simulink library "Junction_Lib"  (R2019a)
settings: Solver=VariableStepAuto  StartTime=0.0  StopTime=10.0  RelTol=1e-3
settings Model: Creator=martin  LastModifiedBy=martin

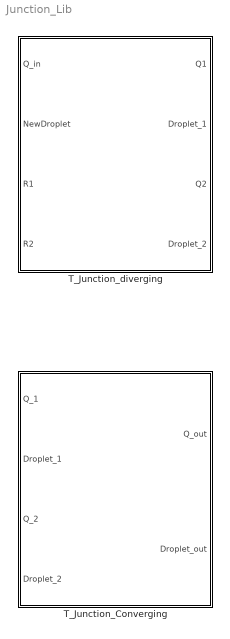
== system Junction_Lib ==
  T_Junction_Converging : Subsystem
  T_Junction_diverging : Subsystem

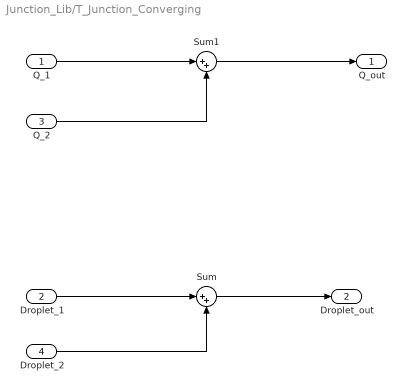
== system Junction_Lib/T_Junction_Converging ==
  Q_1 : Inport
  Droplet_1 : Inport  Port=2
  Q_2 : Inport  Port=3
  Droplet_2 : Inport  Port=4
  Sum : Sum  Inputs=|++
  Sum1 : Sum  Inputs=|++
  Q_out : Outport
  Droplet_out : Outport  Port=2
  wires:
  Droplet_1/1 -> Sum/1
  Sum/1 -> Droplet_out/1
  Droplet_2/1 -> Sum/2
  Q_1/1 -> Sum1/1
  Sum1/1 -> Q_out/1
  Q_2/1 -> Sum1/2

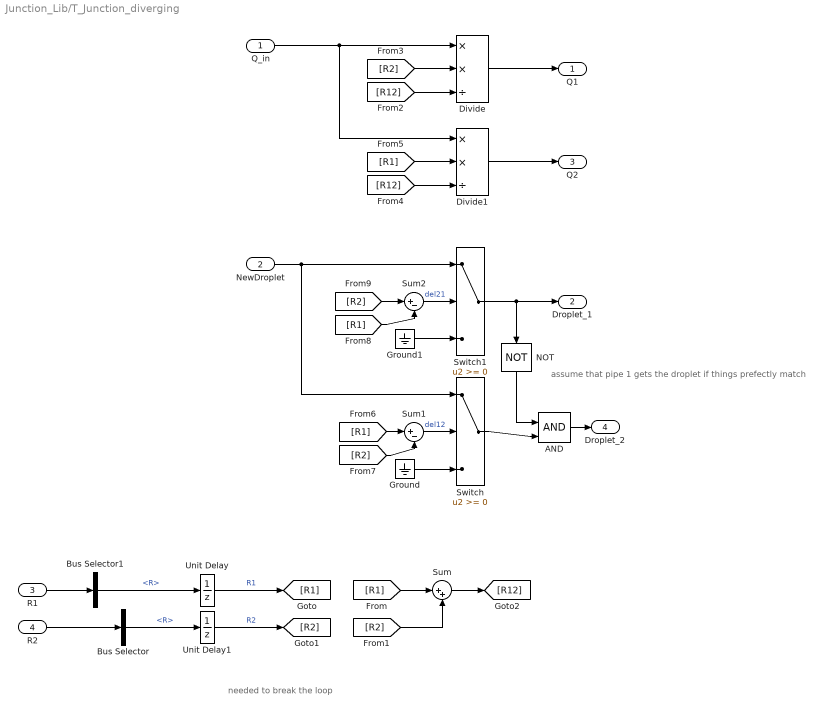
== system Junction_Lib/T_Junction_diverging ==
  note: assume that pipe 1 gets the droplet if things prefectly match
  note: needed to break the loop
  Q_in : Inport
  NewDroplet : Inport  Port=2
  R1 : Inport  Port=3
  R2 : Inport  Port=4
  AND : Logic  IconShape=distinctive  AllPortsSameDT=off  OutDataTypeStr=boolean
  Bus Selector : BusSelector  OutputSignals=R
  Bus Selector1 : BusSelector  OutputSignals=R
  Divide : Product  Inputs=**/
  Divide1 : Product  Inputs=**/
  Ground : Ground
  Ground1 : Ground
  NOT : Logic  Operator=NOT  IconShape=distinctive  AllPortsSameDT=off  OutDataTypeStr=boolean
  Sum : Sum  Inputs=|++
  Sum1 : Sum  Inputs=|+-
  Sum2 : Sum  Inputs=|+-
  Switch : Switch
  Switch1 : Switch
  Unit Delay : UnitDelay  SampleTime=-1  HasFrameUpgradeWarning=on
  Unit Delay1 : UnitDelay  SampleTime=-1  HasFrameUpgradeWarning=on
  Q1 : Outport
  Droplet_1 : Outport  Port=2
  Q2 : Outport  Port=3
  Droplet_2 : Outport  Port=4
  wires:
  Bus Selector/1 -> Unit Delay1/1  "<R>"
  Bus Selector1/1 -> Unit Delay/1  "<R>"
  NOT/1 -> AND/1
  AND/1 -> Droplet_2/1
  [R1] -> Sum2/2
  [R2] -> Sum2/1
  Sum2/1 -> Switch1/2  "del21"
  Switch1/1 -> Droplet_1/1, NOT/1
  NewDroplet/1 -> Switch/1, Switch1/1
  Ground1/1 -> Switch1/3
  Sum1/1 -> Switch/2  "del12"
  [R2] -> Sum1/2
  [R1] -> Sum1/1
  Switch/1 -> AND/2
  Ground/1 -> Switch/3
  Divide/1 -> Q1/1
  Divide1/1 -> Q2/1
  [R12] -> Divide1/3
  [R1] -> Divide1/2
  Q_in/1 -> Divide/1, Divide1/1
  [R2] -> Divide/2
  [R12] -> Divide/3
  Unit Delay1/1 -> [R2]  "R2"
  Unit Delay/1 -> [R1]  "R1"
  Sum/1 -> [R12]
  [R2] -> Sum/2
  [R1] -> Sum/1
  R2/1 -> Bus Selector/1
  R1/1 -> Bus Selector1/1
